simulink model "model_PI_regulator_with_lead"  (Simulink 7.1)
settings: Solver=ode45  StartTime=0.0  StopTime=3000  RelTol=1e-3
libraries: simulink x2
settings Model: Creator=ahp  LastModifiedBy=ahp

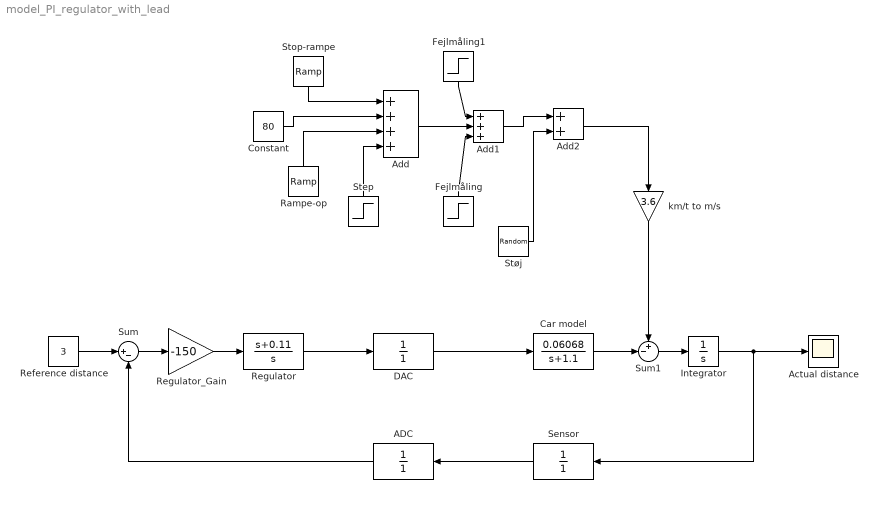
== system model_PI_regulator_with_lead ==
  ADC : TransferFcn  Orientation=left  Denominator=[1]
  Actual distance : Scope
      settings: YMin=2  YMax=4
  Add : Sum  Inputs=++++  OutDataType=sfix(16)  OutScaling=2^-10
  Add1 : Sum  Inputs=+++  OutDataType=sfix(16)  OutScaling=2^-10
  Add2 : Sum  OutDataType=sfix(16)  OutScaling=2^-10
  Car model : TransferFcn  Numerator=[0.06068]  Denominator=[1 1.1]
  Constant : Constant  Value=80  OutDataType=sfix(16)  OutScaling=2^0
  DAC : TransferFcn  Denominator=[1]
  Fejlmåling : Step  Orientation=up  Time=2000  After=-8  SampleTime=0
  Fejlmåling1 : Step  Orientation=down  Time=2010  After=8  SampleTime=0
  Integrator : Integrator
  Rampe-op : simulink/Sources/Ramp  Orientation=up  SystemSampleTime=-1  slope=10/200  start=300  X0=0
  Reference distance : Constant  Value=3  OutDataType=sfix(16)  OutScaling=2^0
  Regulator : TransferFcn  Numerator=[1 0.11]  Denominator=[1 0]
  Regulator_Gain : Gain  Gain=-150  ParameterDataType=sfix(16)  ParameterScaling=2^0  OutDataType=sfix(16)  OutScaling=2^0
  Sensor : TransferFcn  Orientation=left  Denominator=[1]
  Step : Step  Orientation=up  Time=1000  After=-10  SampleTime=0
  Stop-rampe : simulink/Sources/Ramp  Orientation=down  SystemSampleTime=-1  slope=-10/200  start=500  X0=0
  Støj : RandomNumber  Variance=0.05  SampleTime=0
  Sum : Sum  Inputs=|+-  OutDataType=sfix(16)  OutScaling=2^0
  Sum1 : Sum  Inputs=+-|  OutDataType=sfix(16)  OutScaling=2^0
  km/t to m/s : Gain  Orientation=down  Gain=3.6  ParameterDataType=sfix(16)  ParameterScaling=2^0  OutDataType=sfix(16)  OutScaling=2^0
  wires:
  Reference distance/1 -> Sum/1
  Sum/1 -> Regulator_Gain/1
  Car model/1 -> Sum1/2
  Sum1/1 -> Integrator/1
  Integrator/1 -> Actual distance/1, Sensor/1
  ADC/1 -> Sum/2
  Regulator/1 -> DAC/1
  DAC/1 -> Car model/1
  Sensor/1 -> ADC/1
  Regulator_Gain/1 -> Regulator/1
  Step/1 -> Add/4
  Rampe-op/1 -> Add/3
  Constant/1 -> Add/2
  Stop-rampe/1 -> Add/1
  Fejlmåling/1 -> Add1/3
  Add/1 -> Add1/2
  Fejlmåling1/1 -> Add1/1
  Add1/1 -> Add2/1
  Add2/1 -> km/t to m/s/1
  Støj/1 -> Add2/2
  km/t to m/s/1 -> Sum1/1
